simulink model "problem_5"  (R2020a)
settings: Solver=VariableStepAuto  StartTime=0.0  StopTime=10.0  RelTol=1e-3
model workspace (MAT data in the model file):
  C = 1e-05
  R = 10
settings Model: Creator=USER  LastModifiedBy=USER

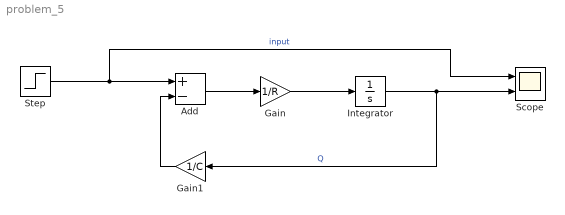
== system problem_5 ==
  Add : Sum  Inputs=+-
  Gain : Gain  Gain=1/R
  Gain1 : Gain  Gain=1/C
  Integrator : Integrator
  Scope : Scope  NumInputPorts=2
  Step : Step  SampleTime=0
  wires:
  Gain1/1 -> Add/2
  Add/1 -> Gain/1
  Integrator/1 -> Gain1/1, Scope/2  "Q"
  Gain/1 -> Integrator/1
  Step/1 -> Scope/1, Add/1  "input"
